simulink model "SubBlockModel"  (R2018b)
settings: Solver=ode45  StartTime=0.0  StopTime=10.0  RelTol=1e-3  EnableMultiTasking=on
PreLoadFcn:
  | load Buses
libraries: CustomLibrary x2
settings Model: Creator=Rose  LastModifiedBy=Rose
settings DataIOCC: LimitDataPoints=on  SaveFormat=Array  SignalLoggingSaveFormat=ModelDataLogs
settings OptimizationCC: DefaultParameterBehavior=Inlined  ExpressionDepthLimit=2147483647  LifeSpan=inf
settings DebuggingCC: UnderspecifiedInitializationDetection=Classic  MergeDetectMultiDrivingBlocksExec=none  SolverPrmCheckMsg=warning  FcnCallInpInsideContextMsg=warning  AllowSymbolicDim=off  StateNameClashWarn=warning  LibraryContextMissingDiagnostic=none  SFUnexpectedBacktrackingDiag=warning  SFNoUnconditionalDefaultTransitionDiag=warning  SFExecutionAtInitializationDiag=none
settings HardwareCC: ProdBitPerPointer=32  ProdBitPerSizeT=32  ProdBitPerPtrDiffT=32  ProdLargestAtomicFloat=None  ProdIntDivRoundTo=Undefined  ProdEndianess=Unspecified  ProdWordSize=32  ProdHWDeviceType=32-bit Generic
settings ModelReferenceCC: PropagateSignalLabelsOutOfModel=off
settings SFSimCC: SimUseLocalCustomCode=off
settings RTWCC: RTWUseLocalCustomCode=off
settings CodeAppCC: StateflowObjectComments=on
settings GRTTargetCC: TargetLangStandard=C89/C90 (ANSI)  GeneratePreprocessorConditionals=Disable all  CombineOutputUpdateFcns=off  GRTInterface=on
settings ConfigComp: CovMetricSettings=dw  CovHtmlReporting=on  CovSaveCumulativeToWorkspaceVar=on  CovSaveSingleToWorkspaceVar=on  CovExternalEMLEnable=off

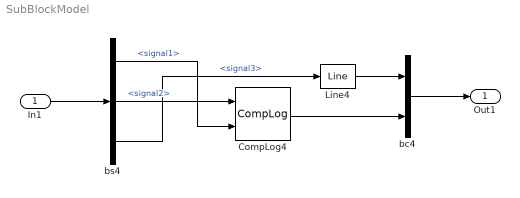
== system SubBlockModel ==
  In1 : Inport  OutDataTypeStr=Bus: Bus_2
  CompLog4 : CustomLibrary/CompLog  SystemSampleTime=-1
  Line4 : CustomLibrary/Line  m=2  b=-1
  bc4 : BusCreator  Inputs=2  OutDataTypeStr=Bus: Bus_1
  bs4 : BusSelector  OutputSignals=signal1,signal2,signal3
  Out1 : Outport  OutDataTypeStr=Bus: Bus_1
  wires:
  In1/1 -> bs4/1
  bc4/1 -> Out1/1
  bs4/2 -> CompLog4/1  "<signal2>"
  bs4/1 -> CompLog4/2  "<signal1>"
  CompLog4/1 -> bc4/2
  bs4/3 -> Line4/1  "<signal3>"
  Line4/1 -> bc4/1
